simulink model "PC_MSFS_STATION"  (R2021b)
settings: Solver=FixedStepAuto  StartTime=0.0  StopTime=2000  FixedStep=0.03  RelTol=1e-3
undefined symbols (not defined in the file): CONTROL, DiscIntNeverNeededParam, f, MODEL, MODEL_INI
libraries: instrumentlib x43, SimConnectToolbox x6, simulink x4
(part 2 of 3)

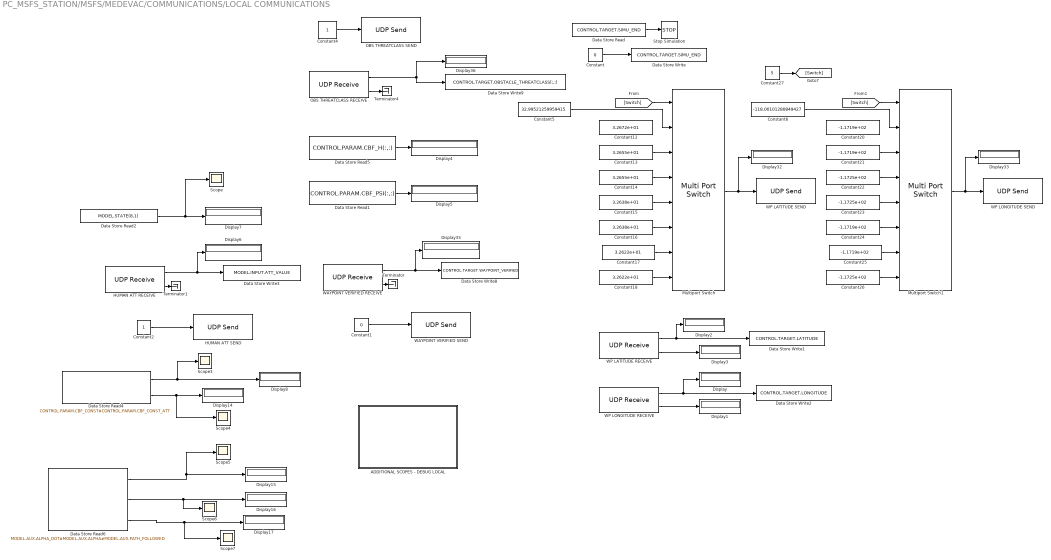
== system PC_MSFS_STATION/MSFS/MEDEVAC/COMMUNICATIONS/LOCAL COMMUNICATIONS ==
  ADDITIONAL SCOPES - DEBUG LOCAL : Subsystem
  Constant : Constant  Value=0  SampleTime=-1
  Constant1 : Constant  Value=0  SampleTime=-1
  Constant12 : Constant  Value=3.2672e+01  SampleTime=0.03
  Constant13 : Constant  Value=3.2655e+01  SampleTime=0.03
  Constant14 : Constant  Value=3.2655e+01  SampleTime=0.03
  Constant15 : Constant  Value=3.2638e+01  SampleTime=0.03
  Constant16 : Constant  Value=3.2638e+01  SampleTime=0.03
  Constant17 : Constant  Value=3.2622e+01  SampleTime=0.03
  Constant18 : Constant  Value=3.2622e+01  SampleTime=0.03
  Constant2 : Constant  SampleTime=-1
  Constant{20..21,24..25} (4 alike) : Constant  Value=-1.1719e+02  SampleTime=0.03
  Constant22 : Constant  Value=-1.1725e+02  SampleTime=0.03
  Constant23 : Constant  Value=-1.1725e+02  SampleTime=0.03
  Constant26 : Constant  Value=-1.1725e+02  SampleTime=0.03
  Constant27 : Constant  Value=5  SampleTime=-1
  Constant4 : Constant  SampleTime=-1
  Constant5 : Constant  Value=32.99521259959415  SampleTime=0.03
  Constant6 : Constant  Value=-118.00101280849427  SampleTime=0.03
  Data Store Read : DataStoreRead  DataStoreName=CONTROL  DataStoreElements=CONTROL.TARGET.SIMU_END  IndexOptions=Index vector (dialog)  Indices=1  OutputSizes=1
  Data Store Read1 : DataStoreRead  DataStoreName=CONTROL  DataStoreElements=CONTROL.PARAM.CBF_PSI(:,:)  IndexOptions=Index vector (dialog)  Indices=1  OutputSizes=1
  Data Store Read2 : DataStoreRead  DataStoreName=MODEL  DataStoreElements=MODEL.STATE(8,1)  IndexOptions=Index vector (dialog)  Indices=1  OutputSizes=1
  Data Store Read4 : DataStoreRead  DataStoreName=CONTROL  DataStoreElements=CONTROL.PARAM.CBF_CONST#CONTROL.PARAM.CBF_CONST_ATT  IndexOptions=Index vector (dialog)  Indices=1  OutputSizes=1
  Data Store Read5 : DataStoreRead  DataStoreName=CONTROL  DataStoreElements=CONTROL.PARAM.CBF_H(:,:)  IndexOptions=Index vector (dialog)  Indices=1  OutputSizes=1
  Data Store Read6 : DataStoreRead  DataStoreName=MODEL  DataStoreElements=MODEL.AUX.ALPHA_DOT#MODEL.AUX.ALPHA#MODEL.AUX.PATH_FOLLOWED  IndexOptions=Index vector (dialog)  Indices=1  OutputSizes=1
  Data Store Write : DataStoreWrite  DataStoreName=CONTROL  DataStoreElements=CONTROL.TARGET.SIMU_END  IndexOptions=Index vector (dialog)  Indices=1  OutputSizes=1
  Data Store Write1 : DataStoreWrite  DataStoreName=CONTROL  DataStoreElements=CONTROL.TARGET.LATITUDE  IndexOptions=Index vector (dialog)  Indices=1  OutputSizes=1
  Data Store Write2 : DataStoreWrite  DataStoreName=CONTROL  DataStoreElements=CONTROL.TARGET.LONGITUDE  IndexOptions=Index vector (dialog)  Indices=1  OutputSizes=1
  Data Store Write3 : DataStoreWrite  DataStoreName=MODEL  DataStoreElements=MODEL.INPUT.ATT_VALUE  IndexOptions=Index vector (dialog)  Indices=1  OutputSizes=1
  Data Store Write8 : DataStoreWrite  DataStoreName=CONTROL  DataStoreElements=CONTROL.TARGET.WAYPOINT_VERIFIED  IndexOptions=Index vector (dialog)  Indices=1  OutputSizes=1
  Data Store Write9 : DataStoreWrite  DataStoreName=CONTROL  DataStoreElements=CONTROL.TARGET.OBSTACLE_THREATCLASS(:,:)  IndexOptions=Index vector (dialog)  Indices=1  OutputSizes=1
  Display{,1..8,14..17,32..33,35..36} (17 alike) : Display
  HUMAN ATT RECEIVE : instrumentlib/UDP Receive  Host=127.0.0.1  Port=7083  LocalPort=7082  EnablePortSharing=off  GetLatestData=off  DataSize="[1  1]"  DataType=double  ASCIIFormatting=%f,  Terminator=LF  ByteOrder=BigEndian  EnableBlockingMode=off  Timeout=10  SampleTime=-1  LocalAddress=127.0.0.1
  HUMAN ATT SEND : instrumentlib/UDP Send  Host=127.0.0.1  Port=7082  LocalPort=7083  EnablePortSharing=off  ByteOrder=BigEndian  OutputDatagramPacketSize=512  EnableBlockingMode=on  LocalAddress=127.0.0.1
  Multiport Switch : MultiPortSwitch  Inputs=7
  Multiport Switch1 : MultiPortSwitch  Inputs=7
  OBS THREATCLASS RECEIVE : instrumentlib/UDP Receive  Host=127.0.0.1  Port=7089  LocalPort=7080  EnablePortSharing=off  GetLatestData=off  DataSize="[1  1]"  DataType=double  ASCIIFormatting=%f,  Terminator=LF  ByteOrder=BigEndian  EnableBlockingMode=off  Timeout=10  SampleTime=-1  LocalAddress=127.0.0.1
  OBS THREATCLASS SEND : instrumentlib/UDP Send  Host=127.0.0.1  Port=7080  LocalPort=7089  EnablePortSharing=off  ByteOrder=BigEndian  OutputDatagramPacketSize=512  EnableBlockingMode=on  LocalAddress=127.0.0.1
  Scope{,3..7} (6 alike) : Scope
  Stop Simulation : Stop
  Terminator : Terminator
  Terminator1 : Terminator
  Terminator4 : Terminator
  WAYPOINT VERIFIED RECEIVE : instrumentlib/UDP Receive  Host=127.0.0.1  Port=7087  LocalPort=7088  EnablePortSharing=off  GetLatestData=off  DataSize="[1  1]"  DataType=double  ASCIIFormatting=%f,  Terminator=LF  ByteOrder=BigEndian  EnableBlockingMode=off  Timeout=10  SampleTime=-1  LocalAddress=127.0.0.1
  WAYPOINT VERIFIED SEND : instrumentlib/UDP Send  Host=127.0.0.1  Port=7088  LocalPort=7087  EnablePortSharing=off  ByteOrder=BigEndian  OutputDatagramPacketSize=512  EnableBlockingMode=on  LocalAddress=127.0.0.1
  WP LATITUDE RECEIVE : instrumentlib/UDP Receive  Host=127.0.0.1  Port=8087  LocalPort=8080  EnablePortSharing=off  GetLatestData=off  DataSize=[1 1]  DataType=double  ASCIIFormatting=%f,  Terminator=LF  ByteOrder=BigEndian  EnableBlockingMode=off  Timeout=10  SampleTime=-1  LocalAddress=127.0.0.1
  WP LATITUDE SEND : instrumentlib/UDP Send  Host=127.0.0.1  Port=8080  LocalPort=8087  EnablePortSharing=off  ByteOrder=BigEndian  OutputDatagramPacketSize=512  EnableBlockingMode=on  LocalAddress=127.0.0.1
  WP LONGITUDE RECEIVE : instrumentlib/UDP Receive  Host=127.0.0.1  Port=8089  LocalPort=8088  EnablePortSharing=off  GetLatestData=off  DataSize=[1 1]  DataType=double  ASCIIFormatting=%f,  Terminator=LF  ByteOrder=BigEndian  EnableBlockingMode=off  Timeout=10  SampleTime=-1  LocalAddress=127.0.0.1
  WP LONGITUDE SEND : instrumentlib/UDP Send  Host=127.0.0.1  Port=8088  LocalPort=8089  EnablePortSharing=off  ByteOrder=BigEndian  OutputDatagramPacketSize=512  EnableBlockingMode=on  LocalAddress=127.0.0.1
  wires:
  Constant6/1 -> Multiport Switch1/2
  Constant5/1 -> Multiport Switch/2
  Constant4/1 -> OBS THREATCLASS SEND/1
  OBS THREATCLASS RECEIVE/2 -> Terminator4/1
  OBS THREATCLASS RECEIVE/1 -> Data Store Write9/1, Display36/1
  Constant27/1 -> [Switch]
  [Switch] -> Multiport Switch1/1
  Constant21/1 -> Multiport Switch1/3
  Constant22/1 -> Multiport Switch1/4
  Constant23/1 -> Multiport Switch1/5
  Constant24/1 -> Multiport Switch1/6
  Constant25/1 -> Multiport Switch1/7
  Constant26/1 -> Multiport Switch1/8
  Multiport Switch1/1 -> Display33/1, WP LONGITUDE SEND/1
  Multiport Switch/1 -> Display32/1, WP LATITUDE SEND/1
  Constant18/1 -> Multiport Switch/8
  Constant17/1 -> Multiport Switch/7
  Constant16/1 -> Multiport Switch/6
  Constant15/1 -> Multiport Switch/5
  Constant14/1 -> Multiport Switch/4
  Constant13/1 -> Multiport Switch/3
  [Switch] -> Multiport Switch/1
  Constant/1 -> Data Store Write/1
  Data Store Read/1 -> Stop Simulation/1
  WP LONGITUDE RECEIVE/2 -> Display1/1
  WP LONGITUDE RECEIVE/1 -> Display/1, Data Store Write2/1
  WP LATITUDE RECEIVE/1 -> Data Store Write1/1, Display2/1
  WP LATITUDE RECEIVE/2 -> Display3/1
  Data Store Read5/1 -> Display4/1
  Data Store Read1/1 -> Display5/1
  WAYPOINT VERIFIED RECEIVE/1 -> Display35/1, Data Store Write8/1
  WAYPOINT VERIFIED RECEIVE/2 -> Terminator/1
  Constant1/1 -> WAYPOINT VERIFIED SEND/1
  Constant2/1 -> HUMAN ATT SEND/1
  HUMAN ATT RECEIVE/2 -> Terminator1/1
  HUMAN ATT RECEIVE/1 -> Data Store Write3/1, Display6/1
  Data Store Read2/1 -> Display7/1, Scope/1
  Data Store Read6/1 -> Scope5/1, Display15/1
  Data Store Read4/2 -> Scope4/1, Display14/1
  Data Store Read6/2 -> Display16/1, Scope6/1
  Data Store Read4/1 -> Display8/1, Scope3/1
  Data Store Read6/3 -> Display17/1, Scope7/1

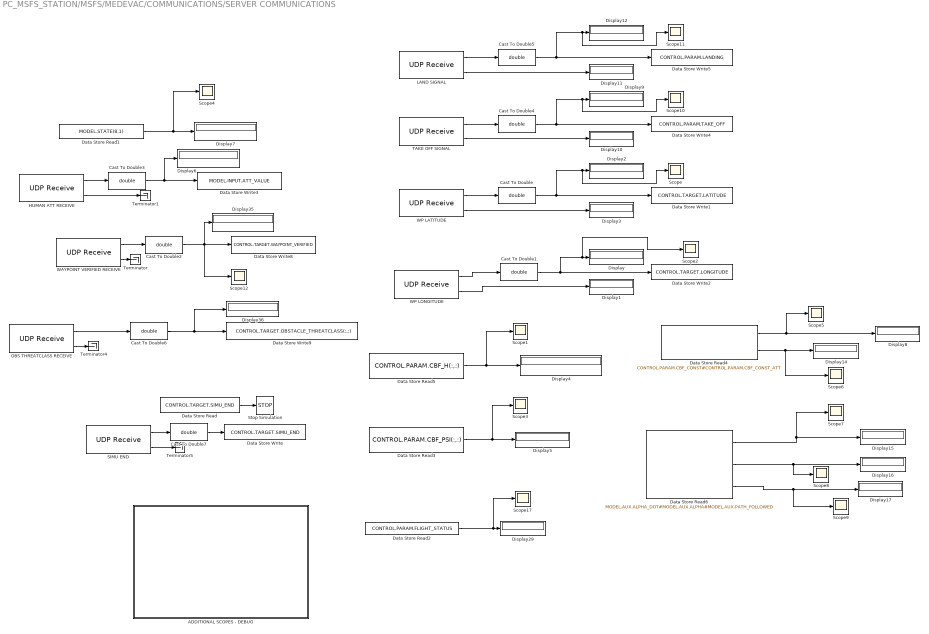
== system PC_MSFS_STATION/MSFS/MEDEVAC/COMMUNICATIONS/SERVER COMMUNICATIONS ==
  ADDITIONAL SCOPES - DEBUG : Subsystem
  Cast To Double{,1..7} (8 alike) : DataTypeConversion  OutDataTypeStr=double
  Data Store Read : DataStoreRead  DataStoreName=CONTROL  DataStoreElements=CONTROL.TARGET.SIMU_END  IndexOptions=Index vector (dialog)  Indices=1  OutputSizes=1
  Data Store Read1 : DataStoreRead  DataStoreName=MODEL  DataStoreElements=MODEL.STATE(8,1)  IndexOptions=Index vector (dialog)  Indices=1  OutputSizes=1
  Data Store Read2 : DataStoreRead  DataStoreName=CONTROL  DataStoreElements=CONTROL.PARAM.FLIGHT_STATUS  IndexOptions=Index vector (dialog)  Indices=1  OutputSizes=1
  Data Store Read3 : DataStoreRead  DataStoreName=CONTROL  DataStoreElements=CONTROL.PARAM.CBF_PSI(:,:)  IndexOptions=Index vector (dialog)  Indices=1  OutputSizes=1
  Data Store Read4 : DataStoreRead  DataStoreName=CONTROL  DataStoreElements=CONTROL.PARAM.CBF_CONST#CONTROL.PARAM.CBF_CONST_ATT  IndexOptions=Index vector (dialog)  Indices=1  OutputSizes=1
  Data Store Read5 : DataStoreRead  DataStoreName=CONTROL  DataStoreElements=CONTROL.PARAM.CBF_H(:,:)  IndexOptions=Index vector (dialog)  Indices=1  OutputSizes=1
  Data Store Read6 : DataStoreRead  DataStoreName=MODEL  DataStoreElements=MODEL.AUX.ALPHA_DOT#MODEL.AUX.ALPHA#MODEL.AUX.PATH_FOLLOWED  IndexOptions=Index vector (dialog)  Indices=1  OutputSizes=1
  Data Store Write : DataStoreWrite  DataStoreName=CONTROL  DataStoreElements=CONTROL.TARGET.SIMU_END  IndexOptions=Index vector (dialog)  Indices=1  OutputSizes=1
  Data Store Write1 : DataStoreWrite  DataStoreName=CONTROL  DataStoreElements=CONTROL.TARGET.LATITUDE  IndexOptions=Index vector (dialog)  Indices=1  OutputSizes=1
  Data Store Write2 : DataStoreWrite  DataStoreName=CONTROL  DataStoreElements=CONTROL.TARGET.LONGITUDE  IndexOptions=Index vector (dialog)  Indices=1  OutputSizes=1
  Data Store Write3 : DataStoreWrite  DataStoreName=MODEL  DataStoreElements=MODEL.INPUT.ATT_VALUE  IndexOptions=Index vector (dialog)  Indices=1  OutputSizes=1
  Data Store Write4 : DataStoreWrite  DataStoreName=CONTROL  DataStoreElements=CONTROL.PARAM.TAKE_OFF  IndexOptions=Index vector (dialog)  Indices=1  OutputSizes=1
  Data Store Write5 : DataStoreWrite  DataStoreName=CONTROL  DataStoreElements=CONTROL.PARAM.LANDING  IndexOptions=Index vector (dialog)  Indices=1  OutputSizes=1
  Data Store Write8 : DataStoreWrite  DataStoreName=CONTROL  DataStoreElements=CONTROL.TARGET.WAYPOINT_VERIFIED  IndexOptions=Index vector (dialog)  Indices=1  OutputSizes=1
  Data Store Write9 : DataStoreWrite  DataStoreName=CONTROL  DataStoreElements=CONTROL.TARGET.OBSTACLE_THREATCLASS(:,:)  IndexOptions=Index vector (dialog)  Indices=1  OutputSizes=1
  Display{,1..12,14..17,29,35..36} (20 alike) : Display
  HUMAN ATT RECEIVE : instrumentlib/UDP Receive  Host=127.0.0.1  Port=7083  LocalPort=7082  EnablePortSharing=off  GetLatestData=off  DataSize="[1  1]"  DataType=double  ASCIIFormatting=%f,  Terminator=LF  ByteOrder=BigEndian  EnableBlockingMode=off  Timeout=10  SampleTime=-1  LocalAddress=127.0.0.1
  LAND SIGNAL : instrumentlib/UDP Receive  Host=127.0.0.1  Port=8081  LocalPort=8086  EnablePortSharing=off  GetLatestData=off  DataSize=[1 1]  DataType=single  ASCIIFormatting=%f,  Terminator=LF  ByteOrder=BigEndian  EnableBlockingMode=off  Timeout=10  SampleTime=-1  LocalAddress=127.0.0.1
  OBS THREATCLASS RECEIVE : instrumentlib/UDP Receive  Host=127.0.0.1  Port=7089  LocalPort=7080  EnablePortSharing=off  GetLatestData=off  DataSize="[1  1]"  DataType=double  ASCIIFormatting=%f,  Terminator=LF  ByteOrder=BigEndian  EnableBlockingMode=off  Timeout=10  SampleTime=-1  LocalAddress=127.0.0.1
  SIMU END : instrumentlib/UDP Receive  Host=127.0.0.1  Port=7086  LocalPort=7084  EnablePortSharing=off  GetLatestData=off  DataSize=[1 1]  DataType=single  ASCIIFormatting=%f,  Terminator=LF  ByteOrder=BigEndian  EnableBlockingMode=off  Timeout=10  SampleTime=-1  LocalAddress=127.0.0.1
  Scope{,1..12,17} (14 alike) : Scope
  Stop Simulation : Stop
  TAKE OFF SIGNAL : instrumentlib/UDP Receive  Host=127.0.0.1  Port=8081  LocalPort=8090  EnablePortSharing=off  GetLatestData=off  DataSize=[1 1]  DataType=single  ASCIIFormatting=%f,  Terminator=LF  ByteOrder=BigEndian  EnableBlockingMode=off  Timeout=10  SampleTime=-1  LocalAddress=127.0.0.1
  Terminator{,1,4..5} (4 alike) : Terminator
  WAYPOINT VERIFIED RECEIVE : instrumentlib/UDP Receive  Host=127.0.0.1  Port=8081  LocalPort=8092  EnablePortSharing=off  GetLatestData=off  DataSize="[1  1]"  DataType=single  ASCIIFormatting=%f,  Terminator=LF  ByteOrder=BigEndian  EnableBlockingMode=off  Timeout=10  SampleTime=-1  LocalAddress=127.0.0.1
  WP LATITUDE : instrumentlib/UDP Receive  Host=127.0.0.1  Port=8081  LocalPort=8080  EnablePortSharing=off  GetLatestData=off  DataSize=[1 1]  DataType=single  ASCIIFormatting=%f,  Terminator=LF  ByteOrder=BigEndian  EnableBlockingMode=off  Timeout=10  SampleTime=-1  LocalAddress=127.0.0.1
  WP LONGITUDE : instrumentlib/UDP Receive  Host=127.0.0.1  Port=8081  LocalPort=8088  EnablePortSharing=off  GetLatestData=off  DataSize=[1 1]  DataType=single  ASCIIFormatting=%f,  Terminator=LF  ByteOrder=BigEndian  EnableBlockingMode=off  Timeout=10  SampleTime=-1  LocalAddress=127.0.0.1
  wires:
  Cast To Double7/1 -> Data Store Write/1
  SIMU END/1 -> Cast To Double7/1
  SIMU END/2 -> Terminator5/1
  Data Store Read/1 -> Stop Simulation/1
  Cast To Double6/1 -> Data Store Write9/1, Display36/1
  OBS THREATCLASS RECEIVE/2 -> Terminator4/1
  OBS THREATCLASS RECEIVE/1 -> Cast To Double6/1
  Cast To Double1/1 -> Data Store Write2/1, Display/1, Scope2/1
  WP LONGITUDE/1 -> Cast To Double1/1
  Cast To Double/1 -> Data Store Write1/1, Display2/1, Scope/1
  WP LATITUDE/1 -> Cast To Double/1
  WP LATITUDE/2 -> Display3/1
  Data Store Read2/1 -> Scope17/1, Display29/1
  WP LONGITUDE/2 -> Display1/1
  WAYPOINT VERIFIED RECEIVE/2 -> Terminator/1
  WAYPOINT VERIFIED RECEIVE/1 -> Cast To Double2/1
  Cast To Double2/1 -> Display35/1, Data Store Write8/1, Scope12/1
  Data Store Read5/1 -> Display4/1, Scope1/1
  Data Store Read3/1 -> Display5/1, Scope3/1
  HUMAN ATT RECEIVE/2 -> Terminator1/1
  Cast To Double3/1 -> Display6/1, Data Store Write3/1
  HUMAN ATT RECEIVE/1 -> Cast To Double3/1
  Data Store Read1/1 -> Display7/1, Scope4/1
  Data Store Read6/1 -> Scope7/1, Display15/1
  Data Store Read4/2 -> Scope6/1, Display14/1
  Data Store Read6/2 -> Display16/1, Scope8/1
  Data Store Read4/1 -> Display8/1, Scope5/1
  Data Store Read6/3 -> Display17/1, Scope9/1
  TAKE OFF SIGNAL/2 -> Display10/1
  TAKE OFF SIGNAL/1 -> Cast To Double4/1
  Cast To Double4/1 -> Scope10/1, Display9/1, Data Store Write4/1
  Cast To Double5/1 -> Data Store Write5/1, Display12/1, Scope11/1
  LAND SIGNAL/1 -> Cast To Double5/1
  LAND SIGNAL/2 -> Display11/1

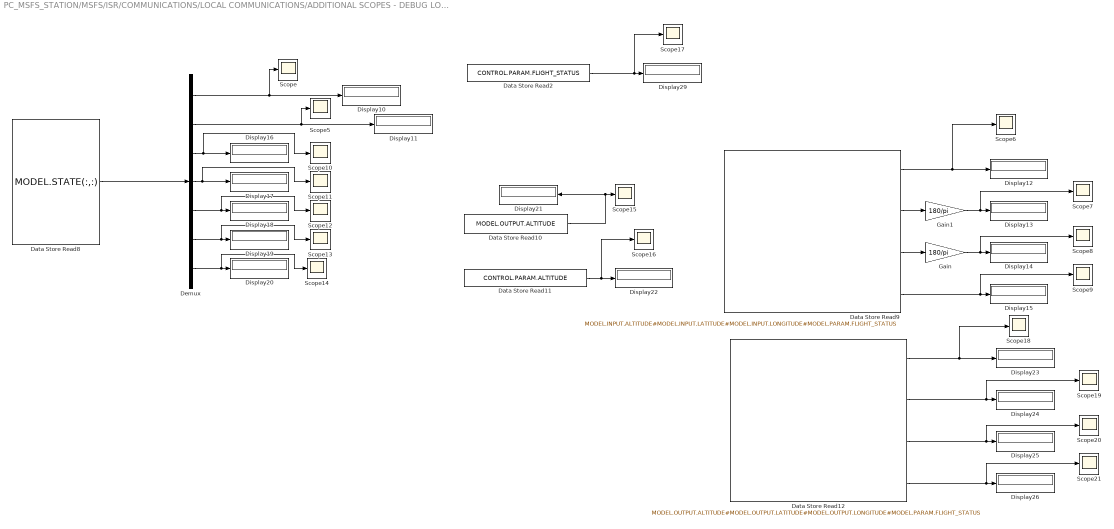
== system PC_MSFS_STATION/MSFS/ISR/COMMUNICATIONS/LOCAL COMMUNICATIONS/ADDITIONAL SCOPES - DEBUG LOCAL ==
  Data Store Read10 : DataStoreRead  DataStoreName=MODEL  DataStoreElements=MODEL.OUTPUT.ALTITUDE  IndexOptions=Index vector (dialog)  Indices=1  OutputSizes=1
  Data Store Read11 : DataStoreRead  DataStoreName=CONTROL  DataStoreElements=CONTROL.PARAM.ALTITUDE  IndexOptions=Index vector (dialog)  Indices=1  OutputSizes=1
  Data Store Read12 : DataStoreRead  DataStoreName=MODEL  DataStoreElements=MODEL.OUTPUT.ALTITUDE#MODEL.OUTPUT.LATITUDE#MODEL.OUTPUT.LONGITUDE#MODEL.PARAM.FLIGHT_STATUS  IndexOptions=Index vector (dialog)  Indices=1  OutputSizes=1
  Data Store Read2 : DataStoreRead  DataStoreName=CONTROL  DataStoreElements=CONTROL.PARAM.FLIGHT_STATUS  IndexOptions=Index vector (dialog)  Indices=1  OutputSizes=1
  Data Store Read8 : DataStoreRead  DataStoreName=MODEL  SampleTime=MODEL_INI.PARAM.SIM_SAMPLING_TIME  DataStoreElements=MODEL.STATE(:,:)  IndexOptions=Index vector (dialog)  Indices=1  OutputSizes=1
  Data Store Read9 : DataStoreRead  DataStoreName=MODEL  DataStoreElements=MODEL.INPUT.ALTITUDE#MODEL.INPUT.LATITUDE#MODEL.INPUT.LONGITUDE#MODEL.PARAM.FLIGHT_STATUS  IndexOptions=Index vector (dialog)  Indices=1  OutputSizes=1
  Demux : Demux  Outputs=7
  Display{10..26,29} (18 alike) : Display
  Gain : Gain  Gain=180/pi
  Gain1 : Gain  Gain=180/pi
  Scope{,5..21} (18 alike) : Scope
  wires:
  Demux/4 -> Scope11/1, Display17/1
  Data Store Read9/3 -> Gain/1
  Data Store Read11/1 -> Scope16/1, Display22/1
  Data Store Read9/2 -> Gain1/1
  Demux/7 -> Scope14/1, Display20/1
  Data Store Read10/1 -> Display21/1, Scope15/1
  Data Store Read8/1 -> Demux/1
  Data Store Read2/1 -> Scope17/1, Display29/1
  Demux/5 -> Scope12/1, Display18/1
  Data Store Read12/2 -> Display24/1, Scope19/1
  Demux/3 -> Scope10/1, Display16/1
  Data Store Read9/4 -> Scope9/1, Display15/1
  Demux/6 -> Scope13/1, Display19/1
  Demux/2 -> Scope5/1, Display11/1
  Data Store Read9/1 -> Display12/1, Scope6/1
  Demux/1 -> Scope/1, Display10/1
  Data Store Read12/1 -> Scope18/1, Display23/1
  Data Store Read12/3 -> Display25/1, Scope20/1
  Data Store Read12/4 -> Display26/1, Scope21/1
  Gain/1 -> Scope8/1, Display14/1
  Gain1/1 -> Scope7/1, Display13/1

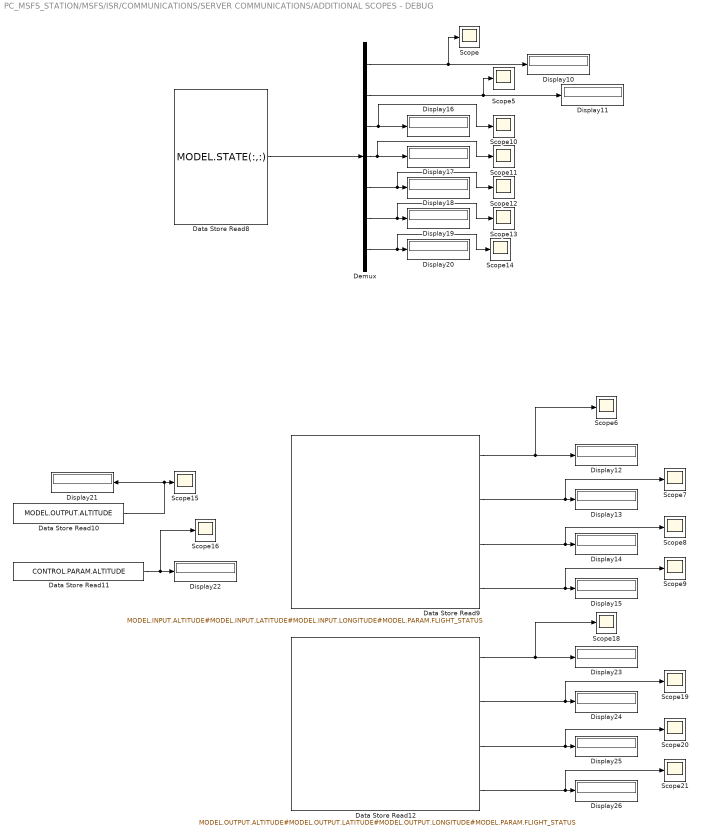
== system PC_MSFS_STATION/MSFS/ISR/COMMUNICATIONS/SERVER COMMUNICATIONS/ADDITIONAL SCOPES - DEBUG ==
  Data Store Read10 : DataStoreRead  DataStoreName=MODEL  DataStoreElements=MODEL.OUTPUT.ALTITUDE  IndexOptions=Index vector (dialog)  Indices=1  OutputSizes=1
  Data Store Read11 : DataStoreRead  DataStoreName=CONTROL  DataStoreElements=CONTROL.PARAM.ALTITUDE  IndexOptions=Index vector (dialog)  Indices=1  OutputSizes=1
  Data Store Read12 : DataStoreRead  DataStoreName=MODEL  DataStoreElements=MODEL.OUTPUT.ALTITUDE#MODEL.OUTPUT.LATITUDE#MODEL.OUTPUT.LONGITUDE#MODEL.PARAM.FLIGHT_STATUS  IndexOptions=Index vector (dialog)  Indices=1  OutputSizes=1
  Data Store Read8 : DataStoreRead  DataStoreName=MODEL  SampleTime=MODEL_INI.PARAM.SIM_SAMPLING_TIME  DataStoreElements=MODEL.STATE(:,:)  IndexOptions=Index vector (dialog)  Indices=1  OutputSizes=1
  Data Store Read9 : DataStoreRead  DataStoreName=MODEL  DataStoreElements=MODEL.INPUT.ALTITUDE#MODEL.INPUT.LATITUDE#MODEL.INPUT.LONGITUDE#MODEL.PARAM.FLIGHT_STATUS  IndexOptions=Index vector (dialog)  Indices=1  OutputSizes=1
  Demux : Demux  Outputs=7
  Display{10..26} (17 alike) : Display
  Scope{,5..16,18..21} (17 alike) : Scope
  wires:
  Data Store Read12/4 -> Scope21/1, Display26/1
  Data Store Read9/2 -> Display13/1, Scope7/1
  Data Store Read9/1 -> Scope6/1, Display12/1
  Demux/4 -> Display17/1, Scope11/1
  Demux/6 -> Display19/1, Scope13/1
  Demux/5 -> Display18/1, Scope12/1
  Demux/7 -> Display20/1, Scope14/1
  Data Store Read9/4 -> Display15/1, Scope9/1
  Data Store Read12/3 -> Scope20/1, Display25/1
  Data Store Read8/1 -> Demux/1
  Data Store Read9/3 -> Display14/1, Scope8/1
  Demux/1 -> Display10/1, Scope/1
  Data Store Read10/1 -> Scope15/1, Display21/1
  Data Store Read11/1 -> Display22/1, Scope16/1
  Demux/2 -> Display11/1, Scope5/1
  Demux/3 -> Display16/1, Scope10/1
  Data Store Read12/1 -> Display23/1, Scope18/1
  Data Store Read12/2 -> Scope19/1, Display24/1

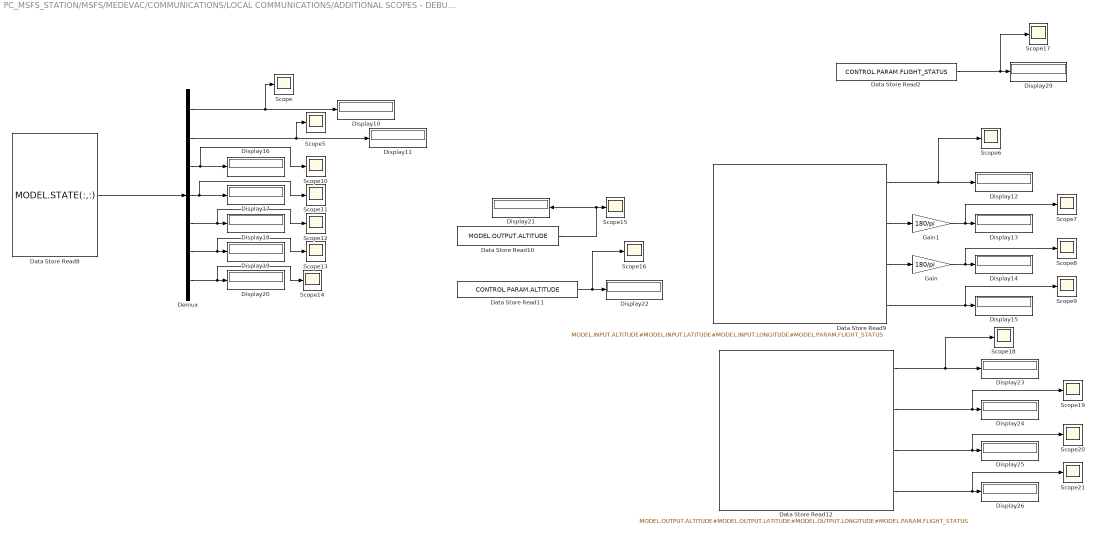
== system PC_MSFS_STATION/MSFS/MEDEVAC/COMMUNICATIONS/LOCAL COMMUNICATIONS/ADDITIONAL SCOPES - DEBUG LOCAL ==
  Data Store Read10 : DataStoreRead  DataStoreName=MODEL  DataStoreElements=MODEL.OUTPUT.ALTITUDE  IndexOptions=Index vector (dialog)  Indices=1  OutputSizes=1
  Data Store Read11 : DataStoreRead  DataStoreName=CONTROL  DataStoreElements=CONTROL.PARAM.ALTITUDE  IndexOptions=Index vector (dialog)  Indices=1  OutputSizes=1
  Data Store Read12 : DataStoreRead  DataStoreName=MODEL  DataStoreElements=MODEL.OUTPUT.ALTITUDE#MODEL.OUTPUT.LATITUDE#MODEL.OUTPUT.LONGITUDE#MODEL.PARAM.FLIGHT_STATUS  IndexOptions=Index vector (dialog)  Indices=1  OutputSizes=1
  Data Store Read2 : DataStoreRead  DataStoreName=CONTROL  DataStoreElements=CONTROL.PARAM.FLIGHT_STATUS  IndexOptions=Index vector (dialog)  Indices=1  OutputSizes=1
  Data Store Read8 : DataStoreRead  DataStoreName=MODEL  SampleTime=MODEL_INI.PARAM.SIM_SAMPLING_TIME  DataStoreElements=MODEL.STATE(:,:)  IndexOptions=Index vector (dialog)  Indices=1  OutputSizes=1
  Data Store Read9 : DataStoreRead  DataStoreName=MODEL  DataStoreElements=MODEL.INPUT.ALTITUDE#MODEL.INPUT.LATITUDE#MODEL.INPUT.LONGITUDE#MODEL.PARAM.FLIGHT_STATUS  IndexOptions=Index vector (dialog)  Indices=1  OutputSizes=1
  Demux : Demux  Outputs=7
  Display{10..26,29} (18 alike) : Display
  Gain : Gain  Gain=180/pi
  Gain1 : Gain  Gain=180/pi
  Scope{,5..21} (18 alike) : Scope
  wires:
  Gain1/1 -> Display13/1, Scope7/1
  Gain/1 -> Display14/1, Scope8/1
  Data Store Read12/4 -> Scope21/1, Display26/1
  Data Store Read12/3 -> Scope20/1, Display25/1
  Data Store Read12/1 -> Display23/1, Scope18/1
  Demux/1 -> Display10/1, Scope/1
  Data Store Read9/1 -> Scope6/1, Display12/1
  Demux/2 -> Display11/1, Scope5/1
  Demux/6 -> Display19/1, Scope13/1
  Data Store Read9/4 -> Display15/1, Scope9/1
  Demux/3 -> Display16/1, Scope10/1
  Data Store Read12/2 -> Scope19/1, Display24/1
  Demux/5 -> Display18/1, Scope12/1
  Data Store Read2/1 -> Display29/1, Scope17/1
  Data Store Read8/1 -> Demux/1
  Data Store Read10/1 -> Scope15/1, Display21/1
  Demux/7 -> Display20/1, Scope14/1
  Data Store Read9/2 -> Gain1/1
  Data Store Read11/1 -> Display22/1, Scope16/1
  Data Store Read9/3 -> Gain/1
  Demux/4 -> Display17/1, Scope11/1

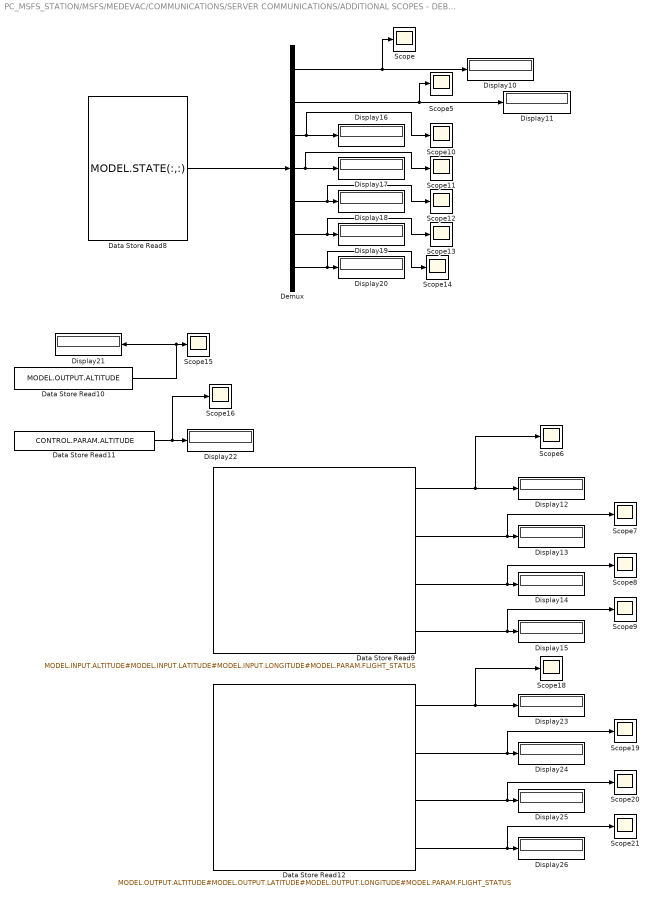
== system PC_MSFS_STATION/MSFS/MEDEVAC/COMMUNICATIONS/SERVER COMMUNICATIONS/ADDITIONAL SCOPES - DEBUG ==
  Data Store Read10 : DataStoreRead  DataStoreName=MODEL  DataStoreElements=MODEL.OUTPUT.ALTITUDE  IndexOptions=Index vector (dialog)  Indices=1  OutputSizes=1
  Data Store Read11 : DataStoreRead  DataStoreName=CONTROL  DataStoreElements=CONTROL.PARAM.ALTITUDE  IndexOptions=Index vector (dialog)  Indices=1  OutputSizes=1
  Data Store Read12 : DataStoreRead  DataStoreName=MODEL  DataStoreElements=MODEL.OUTPUT.ALTITUDE#MODEL.OUTPUT.LATITUDE#MODEL.OUTPUT.LONGITUDE#MODEL.PARAM.FLIGHT_STATUS  IndexOptions=Index vector (dialog)  Indices=1  OutputSizes=1
  Data Store Read8 : DataStoreRead  DataStoreName=MODEL  SampleTime=MODEL_INI.PARAM.SIM_SAMPLING_TIME  DataStoreElements=MODEL.STATE(:,:)  IndexOptions=Index vector (dialog)  Indices=1  OutputSizes=1
  Data Store Read9 : DataStoreRead  DataStoreName=MODEL  DataStoreElements=MODEL.INPUT.ALTITUDE#MODEL.INPUT.LATITUDE#MODEL.INPUT.LONGITUDE#MODEL.PARAM.FLIGHT_STATUS  IndexOptions=Index vector (dialog)  Indices=1  OutputSizes=1
  Demux : Demux  Outputs=7
  Display{10..26} (17 alike) : Display
  Scope{,5..16,18..21} (17 alike) : Scope
  wires:
  Data Store Read12/2 -> Display24/1, Scope19/1
  Data Store Read12/1 -> Scope18/1, Display23/1
  Demux/3 -> Scope10/1, Display16/1
  Demux/2 -> Scope5/1, Display11/1
  Data Store Read11/1 -> Scope16/1, Display22/1
  Data Store Read10/1 -> Display21/1, Scope15/1
  Demux/1 -> Scope/1, Display10/1
  Data Store Read9/3 -> Scope8/1, Display14/1
  Data Store Read8/1 -> Demux/1
  Data Store Read12/3 -> Display25/1, Scope20/1
  Data Store Read9/4 -> Scope9/1, Display15/1
  Demux/7 -> Scope14/1, Display20/1
  Demux/5 -> Scope12/1, Display18/1
  Demux/6 -> Scope13/1, Display19/1
  Demux/4 -> Scope11/1, Display17/1
  Data Store Read9/1 -> Display12/1, Scope6/1
  Data Store Read9/2 -> Scope7/1, Display13/1
  Data Store Read12/4 -> Display26/1, Scope21/1

== matlab function PC_MSFS_STATION/CONTROL/ISR/CONTROL UPDATE ==
  data: CONTROL_IN input; CONTROL output Bus: CONTROL_Bus; STATE input; ALTITUDE_IN input
function CONTROL = CONTROL_UPDATE(CONTROL_IN, STATE, ALTITUDE_IN)
% COPY CONTROL BUS
CONTROL = CONTROL_IN;
CONTROL.PARAM.SIM_TIME = CONTROL.PARAM.SIM_TIME + CONTROL.PARAM.SAMPLING_TIME;
curr_sim_time = CONTROL.PARAM.SIM_TIME;
deltat = CONTROL.PARAM.SAMPLING_TIME;
flight_status = CONTROL.PARAM.FLIGHT_STATUS;
timer = CONTROL.PARAM.TIMER;
sim_control_mode = CONTROL.PARAM.SIM_CONTROL_MODE;
reset_pos_control = CONTROL.PARAM.RESET_POS;
%--------------------------------------------------------------------------
% CONTROL PARAMETERS
%--------------------------------------------------------------------------
% Nominal Control Parameters
kyd = CONTROL.PARAM.NAV_D_1;

% Navigation Variables
%altitude = ALTITUDE_IN;
altitude_control = CONTROL.PARAM.ALTITUDE_REF;
%rho = altitude + 20.902e6;

% Extra Parameters
tau_max = CONTROL.PARAM.TAU_MAX;
%--------------------------------------------------------------------------
% CONTROL TARGETS
%--------------------------------------------------------------------------
simu_end = CONTROL.TARGET.SIMU_END;
target_latitude = CONTROL.TARGET.LATITUDE*pi/180;
target_longitude = CONTROL.TARGET.LONGITUDE*pi/180;
snom = CONTROL.TARGET.VELOCITY;
dist_obstacle = CONTROL.PARAM.DIST_OBSTACLE;
CBF_const = CONTROL.PARAM.CBF_CONST;
human_att_mode = CONTROL.TARGET.HUMAN_ATT_MODE;
%--------------------------------------------------------------------------
% CONTROL OBSTACLES
%--------------------------------------------------------------------------
obs_id = CONTROL.TARGET.OBSTACLE_ID;
obs_lat = CONTROL.TARGET.OBSTACLE_LATITUDE*pi/180;
obs_long = CONTROL.TARGET.OBSTACLE_LONGITUDE*pi/180;
obs_targetclass = CONTROL.TARGET.OBSTACLE_TARGETCLASS; % 1 = AVOID, 0 = FLY OVER
obst_threatclass = CONTROL.TARGET.OBSTACLE_THREATCLASS;
obs_1 = CONTROL.TARGET.OBSTACLE_COORD1;
obs_2 = CONTROL.TARGET.OBSTACLE_COORD2;
%--------------------------------------------------------------------------
% CONTROL CBFS
%--------------------------------------------------------------------------
h = CONTROL.PARAM.CBF_H;
hdot = CONTROL.PARAM.CBF_HDOT;
psi = CONTROL.PARAM.CBF_PSI;
A1_qp = CONTROL.PARAM.CBF_A1QP;
A2_qp = CONTROL.PARAM.CBF_A2QP;
b1_qp = CONTROL.PARAM.CBF_B1QP;


ua_system = CONTROL.OUTPUT.UA;
ualpha_system = CONTROL.OUTPUT.UALPHA;
%--------------------------------------------------------------------------
% SYSTEM CURRENT STATE
%--------------------------------------------------------------------------
% Update Current State
y1 = STATE(1);
y2 = STATE(2);
vy1 = STATE(3);
vy2 = STATE(4);

timer = timer + deltat;

% FLIGHT STATUS 0 = INITIALIZATION
if flight_status == 0
    altitude = ALTITUDE_IN;
    rho = altitude + 20.902e6;
    % VIRTUAL NOMINAL CONTROLLER (tau1, tau2)
    tau1_nom_PD = - kyd*(vy1 - 0);
    tau2_nom_PD = - kyd*(vy2 - 0);
    tau1_applied = tau1_nom_PD;
    tau2_applied = tau2_nom_PD;
    
    if abs(tau1_applied) >= tau_max
        tau1_applied = sign(tau1_applied)*tau_max;
    else
        tau1_applied = tau1_applied;
    end
    
    if abs(tau2_applied) >= tau_max
        tau2_applied = sign(tau2_applied)*tau_max;
    else
        tau2_applied = tau2_applied;
    end
    if curr_sim_time >= 5
        flight_status = 1;
        timer = 0;
    end 

elseif flight_status == 1
    altitude = altitude_control;
    rho = altitude + 20.902e6;
    tau1_nom_PD = - kyd*(vy1 - 0);
    tau2_nom_PD = - kyd*(vy2 - 0);
    tau1_applied = tau1_nom_PD;
    tau2_applied = tau2_nom_PD;
    
    if abs(tau1_applied) >= tau_max
        tau1_applied = sign(tau1_applied)*tau_max;
    else
        tau1_applied = tau1_applied;
    end
    
    if abs(tau2_applied) >= tau_max
        tau2_applied = sign(tau2_applied)*tau_max;
    else
        tau2_applied = tau2_applied;
    end
    if curr_sim_time >= 8
        flight_status = 2;
        timer = 0;
    end

else
    % ON FLIGHT
    %--------------------------------------------------------------------------
    % DERIVATIVE (D) CONTROL
    %--------------------------------------------------------------------------
    altitude = altitude_control;
    rho = altitude + 20.902e6;

    wp1 = rho*cos(target_latitude)*cos(target_longitude);
    wp2 = rho*cos(target_latitude)*sin(target_longitude);
    
    % NOMINAL CONTROLLER
    % System Quadrant
    pos1_PD = wp1 - y1;
    pos2_PD = wp2 - y2;

    if pos1_PD >=0
        % First or fourth quadrant
        if pos2_PD >=0
            %First quadrant
            theta_PD = atan(abs(pos2_PD)/abs(pos1_PD));
        else
            % Fourth quadrant
            %                 theta_PD = 2*pi - atan(abs(pos2_PD)/abs(pos1_PD));
            theta_PD = - atan(abs(pos2_PD)/abs(pos1_PD));
        end
    else
        % Second or third quadrant
        if pos2_PD >=0
            % Second quadrant
            theta_PD = pi - atan(abs(pos2_PD)/abs(pos1_PD));
        else
            % Third quadrant
            theta_PD = pi + atan(abs(pos2_PD)/abs(pos1_PD));
        end
    end

    % New target velocity
    vs1_PD = snom*cos(theta_PD);
    vs2_PD = snom*sin(theta_PD);

    % VIRTUAL NOMINAL CONTROLLER (tau1, tau2)
    tau1_nom_PD = - kyd*(vy1 - vs1_PD);
    tau2_nom_PD = - kyd*(vy2 - vs2_PD);

    if sim_control_mode == 0
        %------------------------------------------------------------------
        % TRACKING ONLY
        %------------------------------------------------------------------
        tau1_applied = tau1_nom_PD;
        tau2_applied = tau2_nom_PD;
    else
        %------------------------------------------------------------------
        % CBF - SAFETY FILTERS: Multiple Obstacles
        %------------------------------------------------------------------

        if (human_att_mode == 1) % Att CBFs
            alpha_val = STATE(8);
            CBF_const_att = CBF_const*alpha_val;
            CONTROL.PARAM.CBF_CONST_ATT = CBF_const_att;
        else % Regular CBFs
            CBF_const_att = CBF_const;
        end
        for i = 1:1:length(obs_id)
            if (obs_id(i) > 0)
                obs_1(i) = rho*cos(obs_lat(i))*cos(obs_long(i));
                obs_2(i) = rho*cos(obs_lat(i))*sin(obs_long(i));

                if (obs_targetclass(i) == 1)
                    dist_obs_scaled = obst_threatclass(i)*dist_obstacle;
                    h(i) = (y1 - obs_1(i))^2 + (y2 - obs_2(i))^2 - dist_obs_scaled^2;
                    hdot(i) = 2*(y1 - obs_1(i))*vy1 + 2*(y2 - obs_2(i))*vy2;
                    psi(i) = hdot(i) + CBF_const_att*h(i);
                    A1_qp(i) = 2*(y1 - obs_1(i));
                    A2_qp(i) = 2*(y2 - obs_2(i));
                    b1_qp(i) = 2*(vy1^2 + vy2^2) + CBF_const_att*hdot(i) + CBF_const_att*psi(i);
                else
                    h(i) = 0;
                    hdot(i) = 0;
                    psi(i) = 0;
                    A1_qp(i) = 0;
                    A2_qp(i) = 0;
                    b1_qp(i) = 0;
                end
            end
        end
           
        A_qp = -[A1_qp(:), A2_qp(:)];
        b_qp = [b1_qp(:)];
        H_qp = 2*[1, 0; 0, 1];
        f_qp = -2*[tau1_nom_PD; tau2_nom_PD];
        x0_qp = [tau1_nom_PD; tau2_nom_PD];
        option_qp = optimoptions('quadprog','Algorithm','active-set','Display','None');
        [tau_applied, fval_qp, exitval_qp] = quadprog(H_qp, double(f_qp), A_qp, b_qp,[],[],[],[],x0_qp,option_qp);
        tau1_applied = tau_applied(1);
        tau2_applied = tau_applied(2);

        CONTROL.PARAM.CBF_H = h(:);
        CONTROL.PARAM.CBF_PSI = psi(:);
    end

    % SATURATE CONTROL INPUT FOR SMOOTH TURNING
    s_system = STATE(5);
    theta_system = STATE(6);
    omega_system = STATE(7);
    p_system = CONTROL.PARAM.DIST_P;
    update_taus = 0;
    ua_system = tau1_applied*cos(theta_system) + tau2_applied*sin(theta_system) + p_system*omega_system^2;
    ualpha_system = -tau1_applied*sin(theta_system)/p_system + tau2_applied*cos(theta_system)/p_system - omega_system*s_system/p_system;
    
%     if (abs(ualpha_system) > 2000)
%         ualpha_system = 2000*sign(ualpha_system);
%     end
%     if (abs(ua_system) > 2000)
%         ua_system = 2000*sign(ua_system);
%         update_taus = 1;
%     end
%     if (update_taus == 1)
%         tau1_applied = ua_system*cos(theta_system) - ualpha_system*p_system*sin(theta_system) - s_system*omega_system*sin(theta_system) - p_system*omega_system^2*cos(theta_system);
%         tau2_applied = ua_system*sin(theta_system) + ualpha_system*p_system*cos(theta_system) + s_system*omega_system*cos(theta_system) - p_system*omega_system^2*sin(theta_system);
%     end
    
    if abs(tau1_applied) >= tau_max
        tau1_applied = sign(tau1_applied)*tau_max;
    else
        tau1_applied = tau1_applied;
    end

    if abs(tau2_applied) >= tau_max
        tau2_applied = sign(tau2_applied)*tau_max;
    else
        tau2_applied = tau2_applied;
    end
    
    
end


%%%%%%%%%%%%%%%%%%%%%%%%%%%%%%%%%%%%%%%%%%%%%%%%%%%%%%%%%%%%%%%%%%%%%%%%%%%
% OUTPUT BUS
%%%%%%%%%%%%%%%%%%%%%%%%%%%%%%%%%%%%%%%%%%%%%%%%%%%%%%%%%%%%%%%%%%%%%%%%%%%
CONTROL.TARGET.SIMU_END = simu_end;
CONTROL.OUTPUT.TAU1 = tau1_applied;
CONTROL.OUTPUT.TAU2 = tau2_applied;

CONTROL.OUTPUT.TAU1_NOM = tau1_nom_PD;
CONTROL.OUTPUT.TAU2_NOM = tau2_nom_PD;

CONTROL.PARAM.FLIGHT_STATUS = flight_status;
CONTROL.PARAM.ALTITUDE = altitude;
CONTROL.PARAM.RHO = rho;
CONTROL.PARAM.TIMER = timer;

CONTROL.OUTPUT.UA = ua_system;
CONTROL.OUTPUT.UALPHA = ualpha_system;

return

== matlab function PC_MSFS_STATION/SYSTEM/ISR/UNICYCLE MODEL ==
  data: STATE input; STATE_DERIVATIVE output; MODEL_IN input; MODEL output Bus: MODEL_Bus
function [STATE_DERIVATIVE,MODEL] = SO_UNICYCLE_MODEL(STATE, MODEL_IN)
% COPY MODEL BUS
MODEL = MODEL_IN;
%--------------------------------------------------------------------------
% SO UNICYCLE PARAMETERS
%--------------------------------------------------------------------------
dist_p = MODEL.PARAM.DISP_P;
%--------------------------------------------------------------------------
% SIMULATION PARAMETERS
%--------------------------------------------------------------------------
flight_status = MODEL.PARAM.FLIGHT_STATUS;
heading_offset = MODEL.PARAM.HEADING_OFFSET;
reset_pos = MODEL.PARAM.RESET_POS;
human_att_mode = MODEL.PARAM.HUMAN_ATT_MODE;
human_att_val = MODEL.INPUT.ATT_VALUE;
if (human_att_val <= 0)
    human_att_val = -1;
end
%--------------------------------------------------------------------------
% EVALUATE FLIGHT STATUS
%--------------------------------------------------------------------------
path_followed = 0;
% att_sat_flag = 0;
if flight_status < 1 % Only reading values from MSFS
    % INITIALIZATION
    theta_long = MODEL.INPUT.LONGITUDE;
    phi_lat = MODEL.INPUT.LATITUDE;
    % altitude = MODEL.INPUT.ALTITUDE;
    altitude = MODEL.OUTPUT.ALTITUDE;
    rho = altitude + 20.902e6;
    % Displaced Point Dynamics Y = {y1, y2, vy1, vy2}
    y1 = rho*cos(phi_lat)*cos(theta_long);
    y2 = rho*cos(phi_lat)*sin(theta_long);
    vy1 = 0;
    vy2 = 0;
    % Center of Mass Dynamics X = {x1, x2, s, theta, omega}
    s = 0;
    theta = 0;
    omega = 0;
    alpha = 1;
    x1 = y1 - dist_p*cos(theta);
    x2 = y2 - dist_p*sin(theta);
else % Reading and writing on MSFS
    %--------------------------------------------------------------------------
    % UPDATE STATE VARIABLES
    %--------------------------------------------------------------------------
    % Displaced Point Dynamics Y = {y1, y2, vy1, vy2}
    y1 = STATE(1);
    y2 = STATE(2);
    vy1 = STATE(3);
    vy2 = STATE(4);
    % Center of Mass Dynamics X = {x1, x2, s, theta, omega}
    s = STATE(5);
    theta = STATE(6);
    omega = STATE(7);
    alpha = STATE(8);
  
    x1 = y1 - dist_p*cos(theta);
    x2 = y2 - dist_p*sin(theta);
    % Update Latitude and Longitude
    altitude = MODEL.OUTPUT.ALTITUDE;
    rho = altitude + 20.902e6;
    if y1 >=0
        % First or fourth quadrant
        if y2 >=0
            %First quadrant
            theta_long = atan(abs(y2)/abs(y1));
        else
            % Fourth quadrant
            %         theta_long = 2*pi - atan(abs(y2)/abs(y1));
            theta_long = - atan(abs(y2)/abs(y1));
        end
    else
        % Second or third quadrant
        if y2 >=0
            % Second quadrant
            theta_long = pi - atan(abs(y2)/abs(y1));
        else
            % Third quadrant
            theta_long = pi + atan(abs(y2)/abs(y1));
        end
    end
%     phi_lat = acos(y1/(rho*cos(theta_long)));
    acosarg = sqrt(y1^2 + y2^2)/rho;
    phi_lat = acos(acosarg);
end
%--------------------------------------------------------------------------
% EVALUATE RESET
%--------------------------------------------------------------------------
if reset_pos == 1
    % Reset Position
    phi_lat = MODEL.PARAM.INIT_LAT; % CENTER OF SEARCH GRID
    theta_long = MODEL.PARAM.INIT_LONG; % CENTER OF SEARCH GRID
    altitude = MODEL.OUTPUT.ALTITUDE;
    rho = altitude + 20.902e6;
    % Displaced Point Dynamics Y = {y1, y2, vy1, vy2}
    y1 = rho*cos(phi_lat)*cos(theta_long);
    y2 = rho*cos(phi_lat)*sin(theta_long);
    vy1 = 0;
    vy2 = 0;
    % Center of Mass Dynamics X = {x1, x2, s, theta, omega}
    s = 0;
    theta = 0;
    omega = 0;
    alpha = 1;
    x1 = y1 - dist_p*cos(theta);
    x2 = y2 - dist_p*sin(theta);
end
%--------------------------------------------------------------------------
% HEADING CONTROL
%--------------------------------------------------------------------------
% CHANGE OF FRAME FROM XYZ TO NED
sinPOS_Lat = sin(phi_lat);
cosPOS_Lat = cos(phi_lat);
sinPOS_Long = sin(theta_long);
cosPOS_Long = cos(theta_long);

Iner_to_NED = zeros(3,3);
Iner_to_NED(1,1) = - sinPOS_Lat*cosPOS_Long;
Iner_to_NED(2,1) = - sinPOS_Long;
Iner_to_NED(3,1) = - cosPOS_Lat*cosPOS_Long;
Iner_to_NED(1,2) = - sinPOS_Lat*sinPOS_Long;
Iner_to_NED(2,2) = cosPOS_Long;
Iner_to_NED(3,2) = - cosPOS_Lat*sinPOS_Long;
Iner_to_NED(1,3) = cosPOS_Lat;
Iner_to_NED(2,3) = 0;
Iner_to_NED(3,3) = - sinPOS_Lat;

NED_vy = Iner_to_NED*[vy1;vy2;0];
NED_vy1 = NED_vy(1); % NORTH
NED_vy2 = NED_vy(2); % EAST
heading_NED = atan2(NED_vy2,NED_vy1) + heading_offset;
heading = atan2(vy2,vy1) + heading_offset;
%--------------------------------------------------------------------------
% INPUTS
%--------------------------------------------------------------------------
tau1 = MODEL.INPUT.TAU1;
tau2 = MODEL.INPUT.TAU2;
%--------------------------------------------------------------------------
% STATE EQUATIONS
%--------------------------------------------------------------------------
y1dot = vy1;
y2dot = vy2;
y1ddot = tau1;
y2ddot = tau2;
sdot = -omega^2*dist_p + tau1*cos(theta) + tau2*sin(theta);
thetadot = omega;
omegadot = 1/dist_p*(omega*s - tau1*sin(theta) + tau2*cos(theta));
if (human_att_mode == 1) % Att CBFs
    alphadot = MODEL.PARAM.ATT_SCALE_FACTOR * human_att_val;
    path_followed =1;
else
    alphadot = 0;
    path_followed = 4;
end
if ((alpha < 1)&&(human_att_val <= 0))
    alphadot = 0;
    alpha = 1;
    path_followed = 2;
end
if ((alpha > 100)&&(human_att_val >=0))
    alphadot = 0;
    alpha = 100;
    path_followed = 3;
end
%--------------------------------------------------------------------------
% STATE DERIVATIVES
%--------------------------------------------------------------------------
STATE_DERIVATIVE = [y1dot; y2dot; y1ddot; y2ddot; sdot; thetadot; omegadot; alphadot];
%%%%%%%%%%%%%%%%%%%%%%%%%%%%%%%%%%%%%%%%%%%%%%%%%%%%%%%%%%%%%%%%%%%%%%%%%%%
% OUTPUT BUS
%%%%%%%%%%%%%%%%%%%%%%%%%%%%%%%%%%%%%%%%%%%%%%%%%%%%%%%%%%%%%%%%%%%%%%%%%%%
MODEL.STATE = [y1 ; y2 ; vy1 ; vy2 ; s ; theta ; omega; alpha];
MODEL.OUTPUT.X1 = x1;
MODEL.OUTPUT.X2 = x2;
MODEL.OUTPUT.X = sqrt(x1^2 + x2^2);
MODEL.OUTPUT.Y = sqrt(y1^2 + y2^2);

MODEL.OUTPUT.LATITUDE = phi_lat;
MODEL.OUTPUT.LONGITUDE = theta_long;
MODEL.OUTPUT.HEADING = heading;
MODEL.OUTPUT.HEADING_NED = heading_NED;

MODEL.AUX.ALPHA_DOT = alphadot;
MODEL.AUX.ALPHA = alpha;
MODEL.AUX.PATH_FOLLOWED = path_followed;
return

== matlab function PC_MSFS_STATION/SYSTEM/MEDEVAC/UNICYCLE MODEL ==
  data: STATE input; STATE_DERIVATIVE output; MODEL_IN input; MODEL output Bus: MODEL_Bus
function [STATE_DERIVATIVE,MODEL] = SO_UNICYCLE_MODEL(STATE, MODEL_IN)
% COPY MODEL BUS
MODEL = MODEL_IN;
%--------------------------------------------------------------------------
% SO UNICYCLE PARAMETERS
%--------------------------------------------------------------------------
dist_p = MODEL.PARAM.DISP_P;
%--------------------------------------------------------------------------
% SIMULATION PARAMETERS
%--------------------------------------------------------------------------
flight_status = MODEL.PARAM.FLIGHT_STATUS;
heading_offset = MODEL.PARAM.HEADING_OFFSET;
reset_pos = MODEL.PARAM.RESET_POS;
first_it_flag = MODEL.PARAM.FIRST_IT;
human_att_mode = MODEL.PARAM.HUMAN_ATT_MODE;
att_sat_flag = MODEL.PARAM.ATT_SAT_FLAG;
%--------------------------------------------------------------------------
% SAVE OLD GEOMETRIC COORDINATES
%--------------------------------------------------------------------------
prev_lat = MODEL.OUTPUT.LATITUDE;
prev_long = MODEL.OUTPUT.LONGITUDE;
prev_head = MODEL.OUTPUT.HEADING;
prev_head_NED = MODEL.OUTPUT.HEADING_NED;
%--------------------------------------------------------------------------
% EVALUATE FLIGHT STATUS
%--------------------------------------------------------------------------
path_followed = 0;
if flight_status < 1 % Only reading values from MSFS
    if (first_it_flag < 2)
        MODEL.PARAM.INIT_LAT = MODEL.INPUT.LATITUDE; % CENTER OF SEARCH GRID
        MODEL.PARAM.INIT_LONG = MODEL.INPUT.LONGITUDE;
        first_it_flag = first_it_flag + 1;
    end
    % INITIALIZATION
    theta_long = MODEL.INPUT.LONGITUDE;
    phi_lat = MODEL.INPUT.LATITUDE;
    % altitude = MODEL.INPUT.ALTITUDE;
    altitude = MODEL.OUTPUT.ALTITUDE;
    rho = altitude + 20.902e6;
    % Displaced Point Dynamics Y = {y1, y2, vy1, vy2}
    y1 = rho*cos(phi_lat)*cos(theta_long);
    y2 = rho*cos(phi_lat)*sin(theta_long);
    vy1 = 0;
    vy2 = 0;
    % Center of Mass Dynamics X = {x1, x2, s, theta, omega}
    s = 0;
    theta = 0;
    omega = 0;
    alpha = 1;
    x1 = y1 - dist_p*cos(theta);
    x2 = y2 - dist_p*sin(theta);
else % Reading and writing on MSFS
    %--------------------------------------------------------------------------
    % UPDATE STATE VARIABLES
    %--------------------------------------------------------------------------
    % Displaced Point Dynamics Y = {y1, y2, vy1, vy2}
    y1 = STATE(1);
    y2 = STATE(2);
    vy1 = STATE(3);
    vy2 = STATE(4);
    % Center of Mass Dynamics X = {x1, x2, s, theta, omega}
    s = STATE(5);
    theta = STATE(6);
    omega = STATE(7);
    alpha = STATE(8);
   
    x1 = y1 - dist_p*cos(theta);
    x2 = y2 - dist_p*sin(theta);
    % Update Latitude and Longitude
    altitude = MODEL.OUTPUT.ALTITUDE;
    rho = altitude + 20.902e6;
    theta_long = atan2(y2,y1);
%     if y1 >=0
%         % First or fourth quadrant
%         if y2 >=0
%             %First quadrant
%             theta_long = atan(abs(y2)/abs(y1));
%         else
%             % Fourth quadrant
%             %         theta_long = 2*pi - atan(abs(y2)/abs(y1));
%             theta_long = - atan(abs(y2)/abs(y1));
%         end
%     else
%         % Second or third quadrant
%         if y2 >=0
%             % Second quadrant
%             theta_long = pi - atan(abs(y2)/abs(y1));
%         else
%             % Third quadrant
%             theta_long = pi + atan(abs(y2)/abs(y1));
%         end
%     end

%     phi_lat = acos(y1/(rho*cos(theta_long)));
    acosarg = sqrt(y1^2 + y2^2)/rho;
    phi_lat = acos(acosarg);

    if flight_status == 3 %% LANDING (HOVER)
        theta_long = prev_long;
        phi_lat = prev_lat;
    end
end
%--------------------------------------------------------------------------
% EVALUATE RESET
%--------------------------------------------------------------------------
if reset_pos == 1
    % Reset Position
    phi_lat = MODEL.PARAM.INIT_LAT; % CENTER OF SEARCH GRID
    theta_long = MODEL.PARAM.INIT_LONG; % CENTER OF SEARCH GRID
    altitude = MODEL.OUTPUT.ALTITUDE;
    rho = altitude + 20.902e6;
    % Displaced Point Dynamics Y = {y1, y2, vy1, vy2}
    y1 = rho*cos(phi_lat)*cos(theta_long);
    y2 = rho*cos(phi_lat)*sin(theta_long);
    vy1 = 0;
    vy2 = 0;
    % Center of Mass Dynamics X = {x1, x2, s, theta, omega}
    s = 0;
    theta = 0;
    omega = 0;
    alpha = 1;
    x1 = y1 - dist_p*cos(theta);
    x2 = y2 - dist_p*sin(theta);
end
%--------------------------------------------------------------------------
% HEADING CONTROL
%--------------------------------------------------------------------------
% CHANGE OF FRAME FROM XYZ TO NED
sinPOS_Lat = sin(phi_lat);
cosPOS_Lat = cos(phi_lat);
sinPOS_Long = sin(theta_long);
cosPOS_Long = cos(theta_long);

Iner_to_NED = zeros(3,3);
Iner_to_NED(1,1) = - sinPOS_Lat*cosPOS_Long;
Iner_to_NED(2,1) = - sinPOS_Long;
Iner_to_NED(3,1) = - cosPOS_Lat*cosPOS_Long;
Iner_to_NED(1,2) = - sinPOS_Lat*sinPOS_Long;
Iner_to_NED(2,2) = cosPOS_Long;
Iner_to_NED(3,2) = - cosPOS_Lat*sinPOS_Long;
Iner_to_NED(1,3) = cosPOS_Lat;
Iner_to_NED(2,3) = 0;
Iner_to_NED(3,3) = - sinPOS_Lat;

NED_vy = Iner_to_NED*[vy1;vy2;0];
NED_vy1 = NED_vy(1); % NORTH
NED_vy2 = NED_vy(2); % EAST
heading_NED = atan2(NED_vy2,NED_vy1) + heading_offset;
heading = atan2(vy2,vy1) + heading_offset;
%--------------------------------------------------------------------------
% INPUTS
%--------------------------------------------------------------------------
tau1 = MODEL.INPUT.TAU1;
tau2 = MODEL.INPUT.TAU2;
%--------------------------------------------------------------------------
% STATE EQUATIONS
%--------------------------------------------------------------------------
y1dot = vy1;
y2dot = vy2;
y1ddot = tau1;
y2ddot = tau2;
sdot = -omega^2*dist_p + tau1*cos(theta) + tau2*sin(theta);
thetadot = omega;
omegadot = 1/dist_p*(omega*s - tau1*sin(theta) + tau2*cos(theta));
if (human_att_mode == 1) % Att CBFs
    alphadot = MODEL.PARAM.ATT_SCALE_FACTOR * MODEL.INPUT.ATT_VALUE;
    path_followed =1;
else
    alphadot = 0;
    path_followed = 4;
end
if ((alpha < 1)&&(MODEL.INPUT.ATT_VALUE <= 0))
    alphadot = 0;
    alpha = 1;
    path_followed = 2;
end
if ((alpha > 100)&&(MODEL.INPUT.ATT_VALUE >=0))
    alphadot = 0;
    alpha = 100;
    path_followed = 3;
end
%--------------------------------------------------------------------------
% STATE DERIVATIVES
%--------------------------------------------------------------------------
STATE_DERIVATIVE = [y1dot; y2dot; y1ddot; y2ddot; sdot; thetadot; omegadot; alphadot];
%%%%%%%%%%%%%%%%%%%%%%%%%%%%%%%%%%%%%%%%%%%%%%%%%%%%%%%%%%%%%%%%%%%%%%%%%%%
% OUTPUT BUS
%%%%%%%%%%%%%%%%%%%%%%%%%%%%%%%%%%%%%%%%%%%%%%%%%%%%%%%%%%%%%%%%%%%%%%%%%%%
MODEL.STATE = [y1 ; y2 ; vy1 ; vy2 ; s ; theta ; omega; alpha];
MODEL.OUTPUT.X1 = x1;
MODEL.OUTPUT.X2 = x2;
MODEL.OUTPUT.X = sqrt(x1^2 + x2^2);
MODEL.OUTPUT.Y = sqrt(y1^2 + y2^2);

MODEL.OUTPUT.LATITUDE = phi_lat;
MODEL.OUTPUT.LONGITUDE = theta_long;
MODEL.OUTPUT.HEADING = heading;
MODEL.OUTPUT.HEADING_NED = heading_NED;
MODEL.PARAM.FIRST_IT = first_it_flag;
MODEL.PARAM.ATT_SAT_FLAG = att_sat_flag;

MODEL.AUX.ALPHA_DOT = alphadot;
MODEL.AUX.ALPHA = alpha;
MODEL.AUX.PATH_FOLLOWED = path_followed;
return
